simulink model "openloop_model_noweights"  (R2024a)
settings: Solver=VariableStepAuto  StartTime=0.0  StopTime=10.0  RelTol=1e-3
values from neighbouring files (symbols this model uses):
  Plant2 = ulinearize('chaser_target_slosh')    [main.m]
libraries: cstblocks x4, RCTblocks x1
settings Model: Creator=T.FORMOSA  LastModifiedBy=r.de-oliveira
settings SolverCC: AlgebraicLoopSolver=TrustRegion
settings DebuggingCC: AlgebraicLoopMsg=none  UnconnectedInputMsg=warning  UnconnectedOutputMsg=warning  UnconnectedLineMsg=warning  ArithmeticOperatorsInVariantConditions=warning
settings ModelReferenceCC: EnableRefExpFcnMdlSchedulingChecks=on
settings SFSimCC: CustomCodeUndefinedFunction=UseInterfaceOnly
settings RTWCC: GPUComputeCapability=3.5  DLArmComputeVersion=19.05

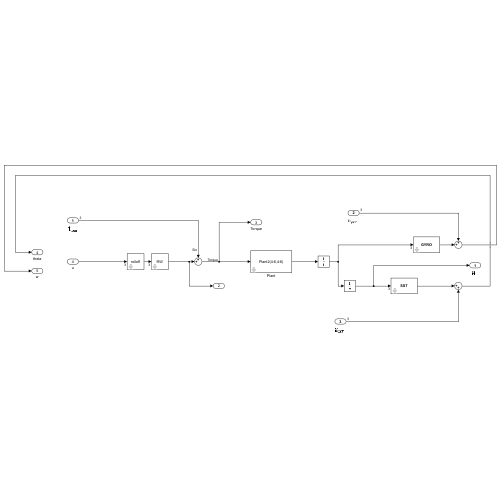
[thumbnail: Simulink's stored preview of the top-level diagram]
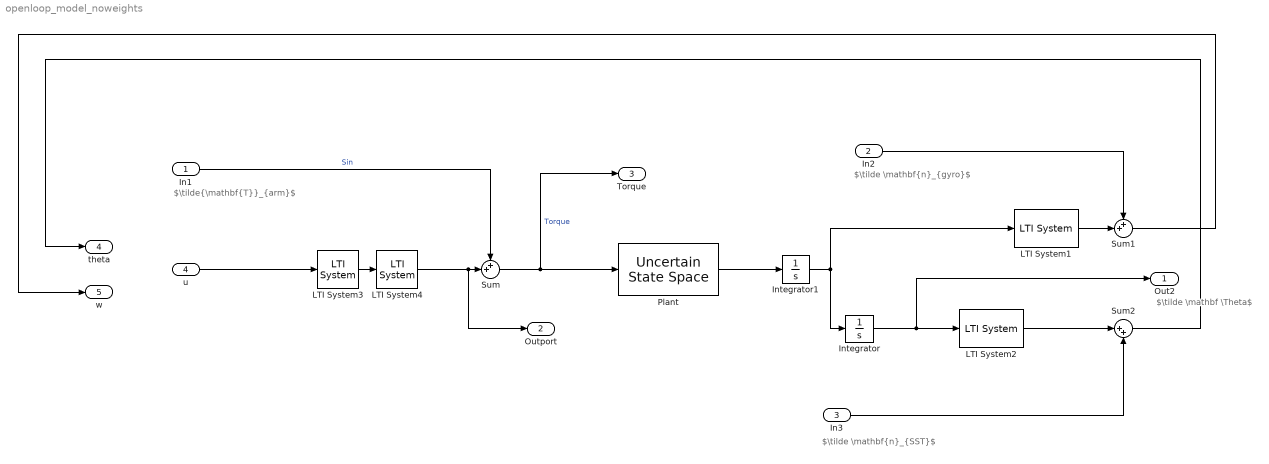
== system openloop_model_noweights ==
  note: $\tilde \mathbf{n}_{SST}$
  note: $\tilde \mathbf{n}_{gyro}$
  note: $\tilde \mathbf \Theta$
  note: $\tilde{\mathbf{T}}_{arm}$
  In1 : Inport  PortDimensions=3
  In2 : Inport  Port=2  PortDimensions=3
  In3 : Inport  Port=3  PortDimensions=3
  u : Inport  Port=4
  Integrator : Integrator
  Integrator1 : Integrator
  LTI System1 : cstblocks/LTI System  sys=GYRO  IC=[]  PadeOrder=0
  LTI System2 : cstblocks/LTI System  sys=SST  IC=[]  PadeOrder=0
  LTI System3 : cstblocks/LTI System  sys=rolloff  IC=[]  PadeOrder=0
  LTI System4 : cstblocks/LTI System  sys=RW  IC=[]  PadeOrder=0
  Plant : RCTblocks/Uncertain State Space  Tag=USS  SCDEnableBlockLinearizationSpecification=on  USystem=Plant2(4:6,4:6)  UValue=[]  X0=[]  uX0=[]
  Sum : Sum  Inputs=++|
  Sum1 : Sum  Inputs=++|
  Sum2 : Sum  Inputs=|++
  Out2 : Outport  VectorParamsAs1DForOutWhenUnconnected=off
  Outport : Outport  Port=2
  Torque : Outport  Port=3
  theta : Outport  Port=4
  w : Outport  Port=5
  wires:
  Integrator1/1 -> LTI System1/1, Integrator/1
  LTI System1/1 -> Sum1/2
  Sum2/1 -> theta/1
  LTI System2/1 -> Sum2/1
  Integrator/1 -> Out2/1, LTI System2/1
  Sum1/1 -> w/1
  Plant/1 -> Integrator1/1
  In2/1 -> Sum1/1
  In3/1 -> Sum2/2
  LTI System3/1 -> LTI System4/1
  LTI System4/1 -> Outport/1, Sum/2
  u/1 -> LTI System3/1
  Sum/1 -> Torque/1, Plant/1  "Torque"
  In1/1 -> Sum/1  "Sin"
